simulink model "lift"  (R2020b)
settings: Solver=VariableStepAuto  StartTime=0.0  StopTime=10.0  RelTol=1e-3
settings Model: EnablePacing=on  PacingRate=0.100000  Creator=Abhinav dixit  LastModifiedBy=Abhinav dixit

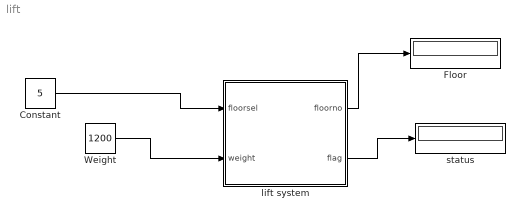
== system lift ==
  Constant : Constant  Value=5
  Floor : Display
  Weight : Constant  Value=1200
  lift system : Stateflow chart  TreatAsAtomicUnit=on
  status : Display
  wires:
  lift system/1(floorno) -> Floor/1
  lift system/2(flag) -> status/1
  Constant/1 -> lift system/1(floorsel)
  Weight/1 -> lift system/2(weight)

== stateflow chart lift/lift system ==
  state check [parallel]
    during:
    overload(weight);
    settings: executionOrder=1
  state LiftMaster [parallel]
    en:
    flag=0;
    settings: executionOrder=2
    state LiftON
      (history)
      state Ground
        entry:
        flag=1;
        during:
        floorno=0;
        floor(floorno);
        exit:
        flag=0;
      state First
        entry:
        flag=1;
        during:
        floorno=1;
        floor(floorno);
        exit:
        flag=0;
      state Third
        entry:
        flag=1;
        during:
        floorno=3;
        floor(floorno)
        exit:
        flag=0;
      state Second
        entry:
        flag=1;
        during:
        floorno=2
        floor(floorno);
        exit:
        flag=0;
      state Fifth
        entry:
        flag=1;
        during:
        floorno=5;
        floor(floorno)
        exit:
        flag=0;
      state Fourth
        entry:
        flag=1;
        during:
        floorno=4;
        floor(floorno)
        exit:
        flag=0;
      (default) -> Ground
      Third -> Fourth [order 2] : up
      Ground -> First : up
      Second -> Third [order 2] : up
      First -> Second [order 1] : up
      Fourth -> Fifth [order 2] : up
      Fifth -> Fourth : down
      First -> Ground [order 2] : down
      Third -> Second [order 1] : down
      Second -> First [order 1] : down
      Fourth -> Third [order 1] : down
    state LiftOFF
      entry:
      flag=0;
    (default) -> LiftON
    LiftON -> LiftOFF : [signal==0]
    LiftOFF -> LiftON : [signal==1]
  state floor(c) [function]
    (default) -> (junction 48)
    (junction 48) -> (junction 52) [order 1] : [floorsel>c]{send(up);
        | disp('LiftGoingUp');}
    (junction 48) -> (junction 51) [order 2] : [floorsel<c]{send(down);
        | disp('LiftGoingDown');}
    (junction 48) -> (junction 55) [order 3] : [floorsel==c]{
        | disp('LiftAlreadyOnFloor');}
    (junction 52) -> (junction 55)
    (junction 51) -> (junction 55)
  state overload(w) [function]
    (default) -> (junction 104)
    (junction 104) -> (junction 107) [order 1] : [w>1200]
    (junction 104) -> (junction 109) [order 2] : {signal=1;}
    (junction 107) -> (junction 111) : {signal=0;}
    (junction 111) -> (junction 109)
  data: c function_input; w function_input; floorsel input; weight input; floorno output; flag output; signal local =1
  events: up local FUNCTION_CALL_EVENT; down local FUNCTION_CALL_EVENT
